simulink model "keyEventSplitter"  (R2016b)
settings: Solver=VariableStepAuto  StartTime=0.0  StopTime=10.0  RelTol=1e-3
settings Model: DataDictionary=DataDictionary.sldd  Creator=Taeke  LastModifiedBy=Taeke

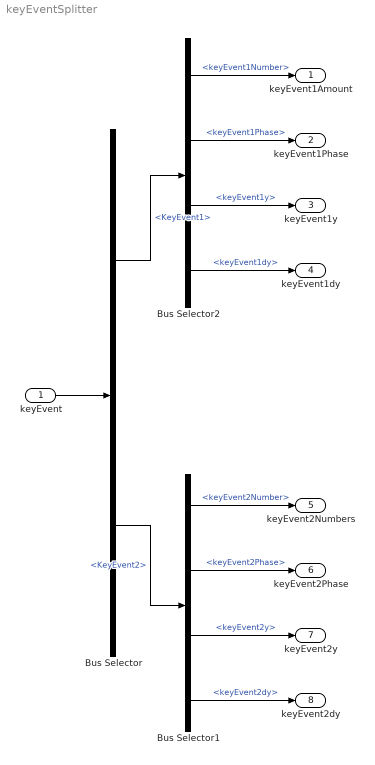
== system keyEventSplitter ==
  keyEvent : Inport  OutDataTypeStr=Bus: keyEventTotal
  Bus Selector : BusSelector  OutputSignals=KeyEvent1,KeyEvent2
  Bus Selector1 : BusSelector  OutputSignals=keyEvent2Number,keyEvent2Phase,keyEvent2y,keyEvent2dy
  Bus Selector2 : BusSelector  OutputSignals=keyEvent1Number,keyEvent1Phase,keyEvent1y,keyEvent1dy
  keyEvent1Amount : Outport
  keyEvent1Phase : Outport  Port=2
  keyEvent1y : Outport  Port=3
  keyEvent1dy : Outport  Port=4
  keyEvent2Numbers : Outport  Port=5
  keyEvent2Phase : Outport  Port=6
  keyEvent2y : Outport  Port=7
  keyEvent2dy : Outport  Port=8
  wires:
  keyEvent/1 -> Bus Selector/1
  Bus Selector1/3 -> keyEvent2y/1  "<keyEvent2y>"
  Bus Selector1/2 -> keyEvent2Phase/1  "<keyEvent2Phase>"
  Bus Selector2/4 -> keyEvent1dy/1  "<keyEvent1dy>"
  Bus Selector2/3 -> keyEvent1y/1  "<keyEvent1y>"
  Bus Selector2/2 -> keyEvent1Phase/1  "<keyEvent1Phase>"
  Bus Selector/1 -> Bus Selector2/1  "<KeyEvent1>"
  Bus Selector/2 -> Bus Selector1/1  "<KeyEvent2>"
  Bus Selector1/4 -> keyEvent2dy/1  "<keyEvent2dy>"
  Bus Selector2/1 -> keyEvent1Amount/1  "<keyEvent1Number>"
  Bus Selector1/1 -> keyEvent2Numbers/1  "<keyEvent2Number>"
